simulink model "Boucle_courant"  (R2017a)
settings: Solver=VariableStepAuto  StartTime=0.0  StopTime=10.0  RelTol=1e-3
values from neighbouring files (symbols this model uses):
  h = 50e-6    (= 5e-05)    [MotorDat_MSTPM1 (1).m]    (also in ParamMinduction0.m; parametres.m = 1e-05)
  Imax = 9.23    [parametres.m]
  J = 0.004    [MotorDat_MSTPM1 (1).m]    (also in ParamMinduction0.m = 0.006; parametres.m = 0.000131)
  K = 55.4e-3    (= 0.0554)    [parametres.m]
  K2 = 3.9789e-4    (= 0.00039789)    [parametres.m]
  kv = 0    [parametres.m]
  L = 1.7e-3    (= 0.0017)    [MotorDat_MSTPM1 (1).m]    (also in parametres.m = 3.08e-05)
  R = 0.13    [MotorDat_MSTPM1 (1).m]    (also in parametres.m = 0.0809)
  Umax = 24    [parametres.m]
undefined symbols (not defined in the file): Kii1, Kpi1
settings Model: Creator=seb  LastModifiedBy=seb

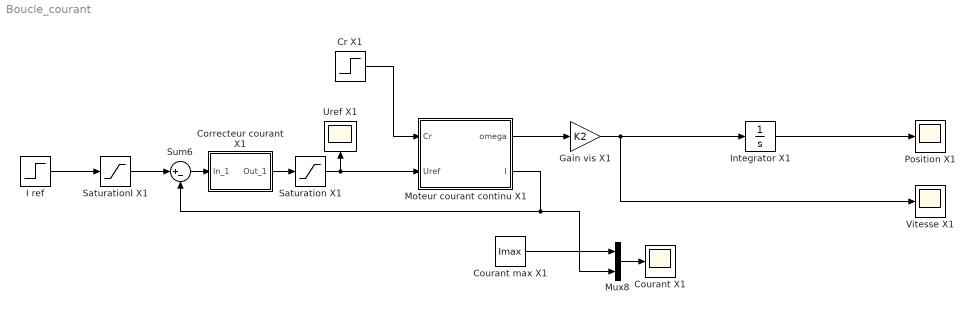
== system Boucle_courant ==
  Correcteur courant X1 : Subsystem  AncestorBlock=simulink_extras/Additional Linear/PID Controller  mask(PID Controller){P=Kpi1, I=Kii1, D=0}
      mask prompts: P "Proportional:"; I "Integral:"; D "Derivative:"
      mask help:
      | Enter expressions for proportional, integral, and derivative terms.
      | P+I/s+Ds
      mask Help: This block implements a PID controller where parameters are entered for the Proportional, Integral and Derivative terms. Unmask this block to see how it works. The derivative term is implemented using a true derivative block.
      mask Display: disp('PI')
  Courant X1 : Scope
  Courant max X1 : Constant  Value=Imax
  Cr X1 : Step  Time=0.30  After=0  SampleTime=0
  Gain vis X1 : Gain  Gain=K2
  I ref : Step  Time=0.2  After=4  SampleTime=0
  Integrator X1 : Integrator
  Moteur courant continu X1 : Subsystem
  Mux8 : Mux  Inputs=2
  Position X1 : Scope
  Saturation X1 : Saturate  UpperLimit=Umax  LowerLimit=-Umax
  SaturationI X1 : Saturate  UpperLimit=Imax  LowerLimit=-Imax
  Sum6 : Sum  Inputs=|+-
  Uref X1 : Scope
  Vitesse X1 : Scope
  wires:
  Correcteur courant X1/1(Out_1) -> Saturation X1/1
  Moteur courant continu X1/2(I) -> Mux8/2, Sum6/2
  Moteur courant continu X1/1(omega) -> Gain vis X1/1
  I ref/1 -> SaturationI X1/1
  Saturation X1/1 -> Moteur courant continu X1/2(Uref), Uref X1/1
  Sum6/1 -> Correcteur courant X1/1(In_1)
  SaturationI X1/1 -> Sum6/1
  Courant max X1/1 -> Mux8/1
  Cr X1/1 -> Moteur courant continu X1/1(Cr)
  Gain vis X1/1 -> Vitesse X1/1, Integrator X1/1
  Integrator X1/1 -> Position X1/1
  Mux8/1 -> Courant X1/1

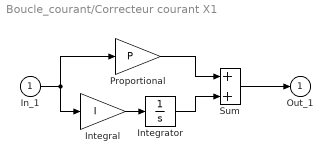
== system Boucle_courant/Correcteur courant X1 ==
  In_1 : Inport
  Integral : Gain  Gain=I  SaturateOnIntegerOverflow=on  OutDataTypeStr=Inherit: Same as input  ParamDataTypeStr=Inherit: Same as input
  Integrator : Integrator  LimitOutput=on  UpperSaturationLimit=Umax  LowerSaturationLimit=-Umax
  Proportional : Gain  Gain=P  SaturateOnIntegerOverflow=on  OutDataTypeStr=Inherit: Same as input  ParamDataTypeStr=Inherit: Same as input
  Sum : Sum  SaturateOnIntegerOverflow=on  InputSameDT=on  OutDataTypeStr=Inherit: Same as first input
  Out_1 : Outport  InitialOutput=0
  wires:
  Proportional/1 -> Sum/1
  In_1/1 -> Proportional/1, Integral/1
  Integrator/1 -> Sum/2
  Integral/1 -> Integrator/1
  Sum/1 -> Out_1/1

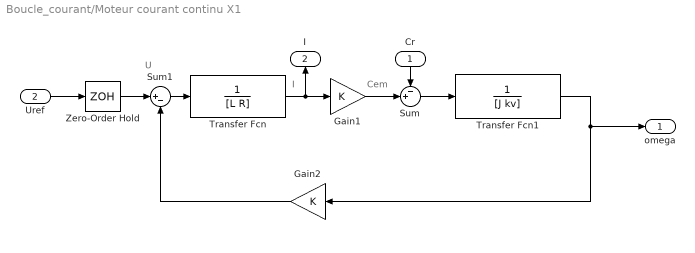
== system Boucle_courant/Moteur courant continu X1 ==
  note: U
  note: I
  note: Cem
  Cr : Inport
  Uref : Inport  Port=2
  Gain1 : Gain  Gain=K
  Gain2 : Gain  Gain=K
  Sum : Sum  Inputs=-+|
  Sum1 : Sum  Inputs=|+-
  Transfer Fcn : TransferFcn  Denominator=[L R]
  Transfer Fcn1 : TransferFcn  Denominator=[J kv]
  Zero-Order Hold : ZeroOrderHold  SampleTime=h
  omega : Outport
  I : Outport  Port=2
  wires:
  Transfer Fcn/1 -> I/1, Gain1/1
  Gain1/1 -> Sum/2
  Sum/1 -> Transfer Fcn1/1
  Transfer Fcn1/1 -> Gain2/1, omega/1
  Sum1/1 -> Transfer Fcn/1
  Gain2/1 -> Sum1/2
  Cr/1 -> Sum/1
  Uref/1 -> Zero-Order Hold/1
  Zero-Order Hold/1 -> Sum1/1
